simulink library "foc_blocks"  (R2020b)
settings: Solver=ode45  StartTime=0.0  StopTime=10.0  RelTol=1e-3  EnableMultiTasking=on
values from neighbouring files (symbols this model uses):
  ClockFrequency = 100    [setup_DF_fixp16_alu_av.m]    (also in setup_sim_DF_fixp16_alu.m; setup_verify_DF_fixp16_alu.m)
  constfractionlengthIn = 10    [setup_DF_fixp16_alu_av.m]    (also in setup_sim_DF_fixp16_alu.m; setup_verify_DF_fixp16_alu.m)
  constwordlengthIn = 16    [setup_DF_fixp16_alu_av.m]    (also in setup_sim_DF_fixp16_alu.m; setup_verify_DF_fixp16_alu.m)
  DSPBASampleTime = FoldingFactor / (ClockFrequency * 1e6)    (= 5e-06)    [setup_DF_fixp16_alu_av.m]    (also in setup_sim_DF_fixp16_alu.m; setup_verify_DF_fixp16_alu.m)
  FoldingFactor = 500    [setup_DF_fixp16_alu_av.m]    (also in setup_sim_DF_fixp16_alu.m; setup_verify_DF_fixp16_alu.m)
undefined symbols (not defined in the file or in its folder): AdvDSPBChannelOutDisplay, dpoly, dspba_ChannelInVis, dspba_ChannelOutVis, dspba_internal_get_channel_ports, evalAionMaskParam, latency, primtype, value, x
libraries: DSPBAPrim x559, AlteraGenericMotorLibrary x20, $bdroot x9, DSPBAUtilities x4, DSPBAControl x4
(part 2 of 6)

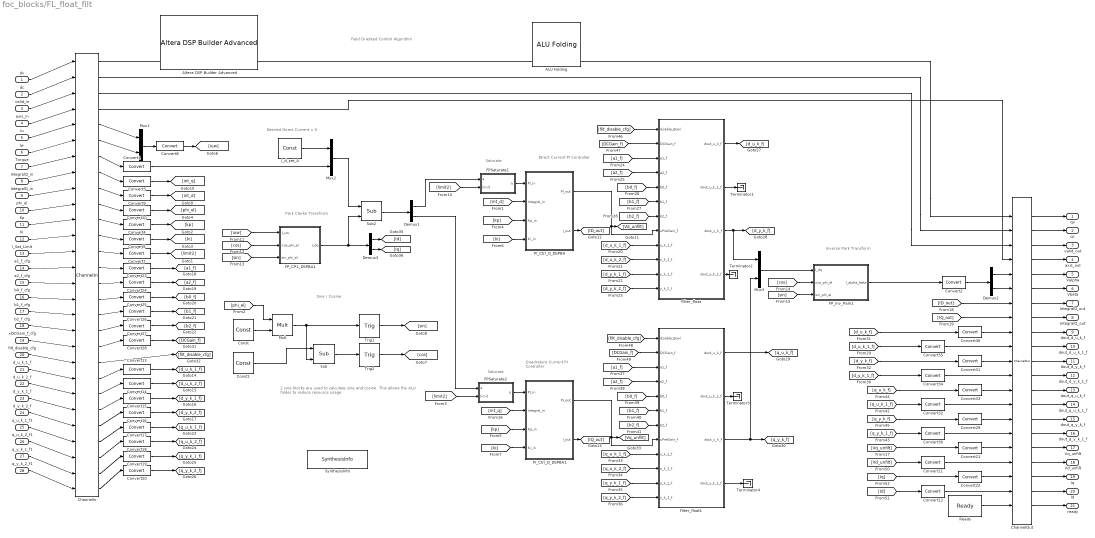
== system foc_blocks/FL_float_filt ==
  note: Quadrature Current
      | PI Controller
  note: Direct Current
      | PI Controller
  note: Desired Direct Current = 0
  note: Inverse Park
      |  Transform
  note: Park Clarke
      |  Transform
  note: Saturate
  note: Saturate
  note: Field Oriented Control Algorithm
  note: Sine / Cosine
  note: 2 sine blocks are used to calculate sine and cosine.
      | This allows the ALU folder to reduce resource usage.
  dv : Inport
  dc : Inport  Port=2
  valid_in : Inport  Port=3
  axis_in : Inport  Port=4
  Iu : Inport  Port=5
  Iw : Inport  Port=6
  Torque : Inport  Port=7
  IntegralQ_in : Inport  Port=8
  IntegralD_in : Inport  Port=9
  phi_el : Inport  Port=10
  Kp : Inport  Port=11
  Ki : Inport  Port=12
  I_Sat_Limit : Inport  Port=13
  a1_f_cfg : Inport  Port=14
  a2_f_cfg : Inport  Port=15
  b0_f_cfg : Inport  Port=16
  b1_f_cfg : Inport  Port=17
  b2_f_cfg : Inport  Port=18
  xDCGain_f_cfg : Inport  Port=19
  filt_disable_cfg : Inport  Port=20
  d_u_k_1_f : Inport  Port=21
  d_u_k_2_f : Inport  Port=22
  d_y_k_1_f : Inport  Port=23
  d_y_k_2_f : Inport  Port=24
  q_u_k_1_f1 : Inport  Port=25
  q_u_k_2_f1 : Inport  Port=26
  q_y_k_1_f1 : Inport  Port=27
  q_y_k_2_f1 : Inport  Port=28
  ALU Folding : DSPBAUtilities/ALU Folding  Description=Enables the new folder. When this block is placed in a subsystem, all primitive subsystems at the level it is placed and below will be passed to the folder. DSP Builder will then generate folded subsystems which can be placed back into the existing design.  version=20130913  genModelFileName=folded_model.xml  sampleRate=SampleRate  numChannels=1  maxLatency=LatencyConstraint  inputFormat=Parallel  outputFormat=Parallel  latchOutputs=off  originalRate=off  hasIdleState=off  padInputs=off  simRate=Clock rate
  Altera DSP Builder Advanced : AlteraGenericMotorLibrary/FP_Cur_Ctrl_DSPBA/Altera DSP Builder Advanced  SystemSampleTime=-1  VariantActivationTime=update diagram  Latency=0  AutoFrameSizeCalculation=off
  ChannelIn : DSPBAPrim/ChannelIn  primtype=channelin  nInputs=dspba_internal_get_channel_ports(gcb)  nOutputs=dspba_internal_get_channel_ports(gcb)  omode=Inherit via internal rule  otype=sfix(16)  scale=2^-15  rndmethod=Unbiased  factor=1  satmethod=Symmetric  shift_vec=[0 1 2 -1]  value=26  inPortNames=['v'; 'c'; '0'; '1'; '2'; '3'; '4'; '5'; '6'; '7'; '8'; '9'; 'A'; 'B'; 'D'; 'E'; 'F'; 'G'; 'H'; 'I'; 'J'; 'K'; 'L'; 'M'; 'N'; 'O'; 'P'; 'Q'; 'R'; 'S'; 'T'; 'U'; 'W'; 'X'; 'Y'; 'Z']  outPortNames=['v'; 'c'; '0'; '1'; '2'; '3'; '4'; '5'; '6'; '7'; '8'; '9'; 'A'; 'B'; 'D'; 'E'; 'F'; 'G'; 'H'; 'I'; 'J'; 'K'; 'L'; 'M'; 'N'; 'O'; 'P'; 'Q'; 'R'; 'S'; 'T'; 'U'; 'W'; 'X'; 'Y'; 'Z']  dspbaimage=dspba_prim.jpg  text=fprintf('In');  style=Optimised  dataSignals=26  foldingEnabled=off  channels=1  sampleRate=ClockFrequency/FoldingFactor  packetBeginPresent=off  packetBeginEnabled=off  visibilities=dspba_ChannelInVis(gcb)  latencyCorrection=0  scheduleOrigin=off  version=20141013
  ChannelOut : DSPBAPrim/ChannelOut  primtype=channelout  nInputs=dspba_internal_get_channel_ports(gcb)  nOutputs=dspba_internal_get_channel_ports(gcb)  omode=Inherit via internal rule  otype=sfix(16)  scale=2^-15  rndmethod=Unbiased  factor=1  satmethod=Symmetric  shift_vec=[0 1 2 -1]  value=19  inPortNames=['v'; 'c'; '0'; '1'; '2'; '3'; '4'; '5'; '6'; '7'; '8'; '9'; 'A'; 'B'; 'D'; 'E'; 'F'; 'G'; 'H'; 'I'; 'J'; 'K'; 'L'; 'M'; 'N'; 'O'; 'P'; 'Q'; 'R'; 'S'; 'T'; 'U'; 'W'; 'X'; 'Y'; 'Z']  outPortNames=['v'; 'c'; '0'; '1'; '2'; '3'; '4'; '5'; '6'; '7'; '8'; '9'; 'A'; 'B'; 'D'; 'E'; 'F'; 'G'; 'H'; 'I'; 'J'; 'K'; 'L'; 'M'; 'N'; 'O'; 'P'; 'Q'; 'R'; 'S'; 'T'; 'U'; 'W'; 'X'; 'Y'; 'Z']  dspbaimage=dspba_prim.jpg  text=fprintf('Out%s', AdvDSPBChannelOutDisplay(latency));  style=Optimised  dataSignals=19  foldingEnabled=off  channels=1  sampleRate=ClockFrequency/FoldingFactor  packetBeginPresent=off  packetBeginEnabled=off  visibilities=dspba_ChannelOutVis(gcb)  latency=173  latencyCorrection=0  version=20141013
  Const : DSPBAPrim/Const  primtype=const  nInputs=0  nOutputs=1  omode=Specify via dialog  otype=fpDT  scale=1  rndmethod=Unbiased  factor=1  satmethod=Symmetric  shift_vec=[0 1 2 -1]  value=2  inPortNames=['+'; '+';]  outPortNames=[' ']  dspbaimage=dspba_prim.jpg  text=fprintf('%s', num2str(value));  style=Optimised  visibilities=8 + 1024  floatPrecision=float26_m17  version=20120820
  Const1 : DSPBAPrim/Const  primtype=const  nInputs=0  nOutputs=1  omode=Specify via dialog  otype=fpDT  scale=1  rndmethod=Unbiased  factor=1  satmethod=Symmetric  shift_vec=[0 1 2 -1]  value=1/2  inPortNames=['+'; '+';]  outPortNames=[' ']  dspbaimage=dspba_prim.jpg  text=fprintf('%s', num2str(value));  style=Optimised  visibilities=8 + 1024  floatPrecision=float26_m17  version=20120820
  Convert{1,3..5,7..10,13..20,23..28} (22 alike) : DSPBAPrim/Convert  primtype=convert  nInputs=1  nOutputs=1  omode=Specify via dialog  otype=fpDT  scale=1  rndmethod=Unbiased  factor=1  satmethod=None  shift_vec=[0 1 2 -1]  value=round([0:255]/17)  inPortNames=[' '; ' ';]  outPortNames=[' '; 'c']  dspbaimage=dspba_prim.jpg  text=fprintf('convert');  style=Optimised  visibilities=8+64+256  clipdetect=off  floatPrecision=float32_m23  advOptions=[]  version=20130211
  Convert{2,11..12,21..22,29..36} (13 alike) : DSPBAPrim/Convert  primtype=convert  nInputs=1  nOutputs=1  omode=single  otype=constOType  scale=constScale  rndmethod=Truncate  factor=1  satmethod=None  shift_vec=[0 1 2 -1]  value=round([0:255]/17)  inPortNames=[' '; ' ';]  outPortNames=[' '; 'c']  dspbaimage=dspba_prim.jpg  text=fprintf('convert');  style=Optimised  visibilities=8+64+256  clipdetect=off  floatPrecision=float32_m23  advOptions=[]  version=20130211
  Demux1 : Demux  Outputs=2
  Demux2 : Demux  Outputs=2
  Demux3 : Demux  Outputs=2
  FPSaturate1 : Subsystem
      mask Display: color('w');fprintf('FP Var Sat\n');port_label('input',1,'a');port_label('input',2,'limit');port_label('output',1,'q');
  FPSaturate2 : Subsystem
      mask Display: color('w');fprintf('FP Var Sat\n');port_label('input',1,'a');port_label('input',2,'limit');port_label('output',1,'q');
  FP_CP1_DSPBA1 : Subsystem  Description=Clarke & Park Transforms
  FP_Inv_Park1 : Subsystem  Description=Inverse Park & Clarke transforms
  Filter_float : Subsystem
  Filter_float1 : Subsystem
  I_d_set_A : DSPBAPrim/Const  primtype=const  nInputs=0  nOutputs=1  omode=Specify via dialog  otype=fpDT  scale=1  rndmethod=Unbiased  factor=1  satmethod=Symmetric  shift_vec=[0 1 2 -1]  value=0  inPortNames=['+'; '+';]  outPortNames=[' ']  dspbaimage=dspba_prim.jpg  text=fprintf('%s', num2str(value));  style=Optimised  visibilities=8 + 1024  floatPrecision=float32_m23  version=20120820
  Mult : DSPBAPrim/Mult  primtype=mult  nInputs=2  nOutputs=1  omode=Inherit via internal rule  otype=sfix(16)  scale=2^-15  rndmethod=Unbiased  factor=1  satmethod=Symmetric  shift_vec=[0 1 2 -1]  value=0  inPortNames=[' '; ' ';]  outPortNames=[' ']  dspbaimage=dspba_prim.jpg  text=fprintf('X');  style=Optimised  visibilities=8+2^18+2^19  floatPrecision=float32_m23  floatRounding=faithful  advOptions=[]  version=20130115
  Mux1 : Mux  Inputs=2
  Mux2 : Mux  Inputs=2
  Mux3 : Mux  Inputs=2
  PI_Ctrl_D_DSPBA : Subsystem
  PI_Ctrl_D_DSPBA1 : Subsystem
  Ready : DSPBAPrim/Ready  primtype=ready  nInputs=0  nOutputs=1  omode=Inherit via internal rule  otype=ufix(1)  scale=2^-0  rndmethod=Unbiased  factor=1  satmethod=Asymmetric  shift_vec=[]  value=1  inPortNames=['']  outPortNames=[' ']  dspbaimage=dspba_prim.jpg  text=fprintf('Ready');  style=Processor  visibilities=0  floatPrecision=float32_m23  version=20131024
  Sub : DSPBAPrim/Sub  primtype=sub  nInputs=2  nOutputs=1  omode=Inherit via internal rule  otype=sfix(16)  scale=2^-15  rndmethod=Unbiased  factor=1  satmethod=Symmetric  shift_vec=[0 1 2 -1]  value=0  inPortNames=['+'; '-';]  outPortNames=[' ']  dspbaimage=dspba_prim.jpg  text=fprintf('-');  style=Optimised  visibilities=8+2^17+2^18  floatRounding=faithful  advOptions=[]  version=20130115
  Sub2 : DSPBAPrim/Sub  primtype=sub  nInputs=2  nOutputs=1  omode=Inherit via internal rule  otype=sfix(16)  scale=2^-15  rndmethod=Unbiased  factor=1  satmethod=Symmetric  shift_vec=[0 1 2 -1]  value=0  inPortNames=['+'; '-';]  outPortNames=[' ']  dspbaimage=dspba_prim.jpg  text=fprintf('-');  style=Optimised  visibilities=8  floatRounding=faithful  advOptions=[]  version=20130115
  SynthesisInfo : DSPBAPrim/SynthesisInfo  primtype=synthinfo  nInputs=0  nOutputs=0  omode=Inherit via internal rule  otype=sfix(16)  scale=2^-15  rndmethod=Truncate  factor=1  satmethod=Symmetric  shift_vec=[0 1 2 -1]  value=99  inPortNames=[' '; ' ';]  outPortNames=[' ']  dspbaimage=dspba_prim_ctrl.jpg  text=fprintf('Style=%s', style);  style=Scheduled  visibilities=32768  constraintInUse=off  constraintRelation=>  constraintLimit=2  bitAccurate=off  version=20150220
  Terminator{1..4} (4 alike) : Terminator
  Trig1 : DSPBAPrim/Trig  primtype=trigfunc  nInputs=1  nOutputs=1  omode=Inherit via internal rule  otype=sfix(16)  scale=2^-15  rndmethod=Unbiased  factor=1  satmethod=Symmetric  shift_vec=[0 1 2 -1]  value=round([0:255]/17)  inPortNames=[' '; ' ';]  outPortNames=[' ']  dspbaimage=dspba_prim_float.jpg  text=fprintf('sin(a)');  style=Optimised  visibilities=2^17+2^18  functionExpr=sin(pi*x)  advOptions=[]  version=20140803
  Trig2 : DSPBAPrim/Trig  primtype=trigfunc  nInputs=1  nOutputs=1  omode=Inherit via internal rule  otype=sfix(16)  scale=2^-15  rndmethod=Unbiased  factor=1  satmethod=Symmetric  shift_vec=[0 1 2 -1]  value=round([0:255]/17)  inPortNames=[' '; ' ';]  outPortNames=[' ']  dspbaimage=dspba_prim_float.jpg  text=fprintf('sin(a)');  style=Optimised  visibilities=2^17+2^18  functionExpr=sin(pi*x)  advOptions=[]  version=20140803
  qv : Outport
  qc : Outport  Port=2
  valid_out : Outport  Port=3
  axis_out : Outport  Port=4
  Valpha : Outport  Port=5
  Vbeta : Outport  Port=6
  IntegralD_out : Outport  Port=7
  IntegralQ_out : Outport  Port=8
  dout_d_u_k_f : Outport  Port=9
  dout_d_u_k_1_f : Outport  Port=10
  dout_d_y_k_f : Outport  Port=11
  dout_d_y_k_1_f : Outport  Port=12
  dout_q_u_k_f : Outport  Port=13
  dout_q_u_k_1_f : Outport  Port=14
  dout_q_y_k_f : Outport  Port=15
  dout_q_y_k_1_f : Outport  Port=16
  Vq_unfilt : Outport  Port=17
  Vd_unfilt : Outport  Port=18
  Iq : Outport  Port=19
  Id : Outport  Port=20
  ready : Outport  Port=21
  wires:
  ChannelIn/1 -> ChannelOut/1
  ChannelIn/2 -> ChannelOut/2
  ChannelIn/5 -> Mux1/1
  ChannelIn/6 -> Mux1/2
  ChannelIn/3 -> ChannelOut/3
  ChannelIn/7 -> Convert1/1
  FPSaturate2/1(q) -> PI_Ctrl_D_DSPBA1/1(PI_in)
  FPSaturate1/1(q) -> PI_Ctrl_D_DSPBA/1(PI_in)
  Mux3/1 -> FP_Inv_Park1/1(I_dq)
  FP_Inv_Park1/1(I_alpha_beta) -> Convert2/1
  Demux2/1 -> ChannelOut/5
  Demux2/2 -> ChannelOut/6
  I_d_set_A/1 -> Mux2/1
  Mux2/1 -> Sub2/1
  Sub2/1 -> Demux1/1
  Demux1/1 -> FPSaturate1/1(a)
  Demux1/2 -> FPSaturate2/1(a)
  ChannelIn/8 -> Convert3/1
  ChannelIn/9 -> Convert9/1
  ChannelIn/10 -> Convert10/1
  ChannelIn/11 -> Convert4/1
  ChannelIn/12 -> Convert5/1
  [int_q] -> PI_Ctrl_D_DSPBA1/2(Integral_in)
  [kp] -> PI_Ctrl_D_DSPBA1/3(Kp_in)
  [ki] -> PI_Ctrl_D_DSPBA1/4(Ki_in)
  [limit2] -> FPSaturate2/2(limit)
  [int_d] -> PI_Ctrl_D_DSPBA/2(Integral_in)
  [kp] -> PI_Ctrl_D_DSPBA/3(Kp_in)
  [ki] -> PI_Ctrl_D_DSPBA/4(Ki_in)
  [limit2] -> FPSaturate1/2(limit)
  [iuw] -> FP_CP1_DSPBA1/1(I_uw)
  [cos] -> FP_CP1_DSPBA1/2(cos_phi_el)
  [sin] -> FP_CP1_DSPBA1/3(sin_phi_el)
  Mux1/1 -> Convert8/1
  [cos] -> FP_Inv_Park1/2(cos_phi_el)
  [sin] -> FP_Inv_Park1/3(sin_phi_el)
  Convert7/1 -> [limit2]
  Convert5/1 -> [ki]
  Convert4/1 -> [kp]
  Convert8/1 -> [iuw]
  Convert1/1 -> Mux2/2
  ChannelIn/4 -> ChannelOut/4
  Convert2/1 -> Demux2/1
  [ID_out] -> ChannelOut/7
  PI_Ctrl_D_DSPBA/2(I_out) -> [ID_out]
  [IQ_out] -> ChannelOut/8
  PI_Ctrl_D_DSPBA1/2(I_out) -> [IQ_out]
  Filter_float/3(dout_y_k_f) -> [d_y_k_f], Mux3/1
  PI_Ctrl_D_DSPBA/1(PI_out) -> Filter_float/8(uPreGain_f), [Vd_unfilt]
  [d_u_k_1_f] -> Filter_float/9(u_k_1_f)
  [d_u_k_2_f] -> Filter_float/10(u_k_2_f)
  [d_y_k_1_f] -> Filter_float/11(y_k_1_f)
  [d_y_k_2_f] -> Filter_float/12(y_k_2_f)
  [b2_f] -> Filter_float/7(b2_f)
  [b1_f] -> Filter_float/6(b1_f)
  [b0_f] -> Filter_float/5(b0_f)
  [a2_f] -> Filter_float/4(a2_f)
  [a1_f] -> Filter_float/3(a1_f)
  Filter_float1/3(dout_y_k_f) -> [q_y_k_f], Mux3/2
  PI_Ctrl_D_DSPBA1/1(PI_out) -> Filter_float1/8(uPreGain_f), [Vq_unfilt]
  [q_u_k_1_f] -> Filter_float1/9(u_k_1_f)
  [q_u_k_2_f] -> Filter_float1/10(u_k_2_f)
  [q_y_k_1_f] -> Filter_float1/11(y_k_1_f)
  [q_y_k_2_f] -> Filter_float1/12(y_k_2_f)
  [b2_f] -> Filter_float1/7(b2_f)
  [b1_f] -> Filter_float1/6(b1_f)
  [b0_f] -> Filter_float1/5(b0_f)
  [a2_f] -> Filter_float1/4(a2_f)
  [a1_f] -> Filter_float1/3(a1_f)
  Filter_float/1(dout_u_k_f) -> [d_u_k_f]
  Filter_float/2(dout_u_k_1_f) -> Terminator1/1
  Filter_float/4(dout_y_k_1_f) -> Terminator2/1
  [filt_disable_cfg] -> Filter_float/1(disable_Bool)
  [DCGain_f] -> Filter_float/2(DCGain_f)
  Filter_float1/4(dout_y_k_1_f) -> Terminator4/1
  Filter_float1/2(dout_u_k_1_f) -> Terminator3/1
  Filter_float1/1(dout_u_k_f) -> [q_u_k_f]
  [filt_disable_cfg] -> Filter_float1/1(disable_Bool)
  [DCGain_f] -> Filter_float1/2(DCGain_f)
  [Vq_unfilt] -> Convert21/1
  [Vd_unfilt] -> Convert11/1
  Ready/1 -> ChannelOut/21
  FP_CP1_DSPBA1/1(I_dq) -> Demux3/1, Sub2/2
  Demux3/1 -> [Id]
  Demux3/2 -> [Iq]
  [Iq] -> Convert22/1
  [Id] -> Convert12/1
  [phi_el] -> Mult/1
  Const/1 -> Mult/2
  Const1/1 -> Sub/1
  Mult/1 -> Trig1/1, Sub/2
  Sub/1 -> Trig2/1
  Trig1/1 -> [sin]
  Trig2/1 -> [cos]
  Convert3/1 -> [int_q]
  Convert9/1 -> [int_d]
  Convert10/1 -> [phi_el]
  Convert22/1 -> ChannelOut/19
  Convert12/1 -> ChannelOut/20
  Convert11/1 -> ChannelOut/18
  Convert21/1 -> ChannelOut/17
  [q_y_k_f] -> Convert29/1
  [d_y_k_f] -> Convert31/1
  Convert23/1 -> [a1_f]
  Convert24/1 -> [a2_f]
  Convert25/1 -> [b0_f]
  Convert26/1 -> [b1_f]
  Convert27/1 -> [b2_f]
  Convert28/1 -> [DCGain_f]
  Convert13/1 -> [d_u_k_1_f]
  Convert14/1 -> [d_u_k_2_f]
  Convert15/1 -> [d_y_k_1_f]
  Convert16/1 -> [d_y_k_2_f]
  Convert17/1 -> [q_u_k_1_f]
  Convert18/1 -> [q_u_k_2_f]
  Convert19/1 -> [q_y_k_1_f]
  Convert20/1 -> [q_y_k_2_f]
  Convert29/1 -> ChannelOut/15
  [q_u_k_f] -> Convert33/1
  Convert31/1 -> ChannelOut/11
  [d_u_k_f] -> Convert36/1
  [q_y_k_1_f] -> Convert30/1
  [q_u_k_1_f] -> Convert32/1
  [d_y_k_1_f] -> Convert34/1
  [d_u_k_1_f] -> Convert35/1
  Convert30/1 -> ChannelOut/16
  Convert32/1 -> ChannelOut/14
  Convert33/1 -> ChannelOut/13
  Convert34/1 -> ChannelOut/12
  Convert35/1 -> ChannelOut/10
  Convert36/1 -> ChannelOut/9
  dv/1 -> ChannelIn/1
  dc/1 -> ChannelIn/2
  valid_in/1 -> ChannelIn/3
  axis_in/1 -> ChannelIn/4
  Iu/1 -> ChannelIn/5
  Iw/1 -> ChannelIn/6
  Torque/1 -> ChannelIn/7
  IntegralQ_in/1 -> ChannelIn/8
  IntegralD_in/1 -> ChannelIn/9
  phi_el/1 -> ChannelIn/10
  Kp/1 -> ChannelIn/11
  Ki/1 -> ChannelIn/12
  ChannelOut/1 -> qv/1
  ChannelOut/2 -> qc/1
  ChannelOut/3 -> valid_out/1
  ChannelOut/4 -> axis_out/1
  ChannelOut/5 -> Valpha/1
  ChannelOut/6 -> Vbeta/1
  ChannelOut/7 -> IntegralD_out/1
  ChannelOut/8 -> IntegralQ_out/1
  ChannelOut/9 -> dout_d_u_k_f/1
  ChannelOut/10 -> dout_d_u_k_1_f/1
  ChannelOut/11 -> dout_d_y_k_f/1
  ChannelOut/12 -> dout_d_y_k_1_f/1
  ChannelOut/13 -> dout_q_u_k_f/1
  ChannelOut/14 -> dout_q_u_k_1_f/1
  ChannelOut/15 -> dout_q_y_k_f/1
  ChannelOut/16 -> dout_q_y_k_1_f/1
  ChannelOut/17 -> Vq_unfilt/1
  ChannelOut/18 -> Vd_unfilt/1
  ChannelOut/19 -> Iq/1
  ChannelOut/20 -> Id/1
  ChannelOut/21 -> ready/1
  I_Sat_Limit/1 -> ChannelIn/13
  a1_f_cfg/1 -> ChannelIn/14
  a2_f_cfg/1 -> ChannelIn/15
  b0_f_cfg/1 -> ChannelIn/16
  b1_f_cfg/1 -> ChannelIn/17
  b2_f_cfg/1 -> ChannelIn/18
  xDCGain_f_cfg/1 -> ChannelIn/19
  filt_disable_cfg/1 -> ChannelIn/20
  d_u_k_1_f/1 -> ChannelIn/21
  d_u_k_2_f/1 -> ChannelIn/22
  d_y_k_1_f/1 -> ChannelIn/23
  d_y_k_2_f/1 -> ChannelIn/24
  q_u_k_1_f1/1 -> ChannelIn/25
  q_u_k_2_f1/1 -> ChannelIn/26
  q_y_k_1_f1/1 -> ChannelIn/27
  q_y_k_2_f1/1 -> ChannelIn/28
  ChannelIn/13 -> Convert7/1
  ChannelIn/14 -> Convert23/1
  ChannelIn/15 -> Convert24/1
  ChannelIn/16 -> Convert25/1
  ChannelIn/17 -> Convert26/1
  ChannelIn/18 -> Convert27/1
  ChannelIn/19 -> Convert28/1
  ChannelIn/20 -> [filt_disable_cfg]
  ChannelIn/21 -> Convert13/1
  ChannelIn/22 -> Convert14/1
  ChannelIn/23 -> Convert15/1
  ChannelIn/24 -> Convert16/1
  ChannelIn/25 -> Convert17/1
  ChannelIn/26 -> Convert18/1
  ChannelIn/27 -> Convert19/1
  ChannelIn/28 -> Convert20/1

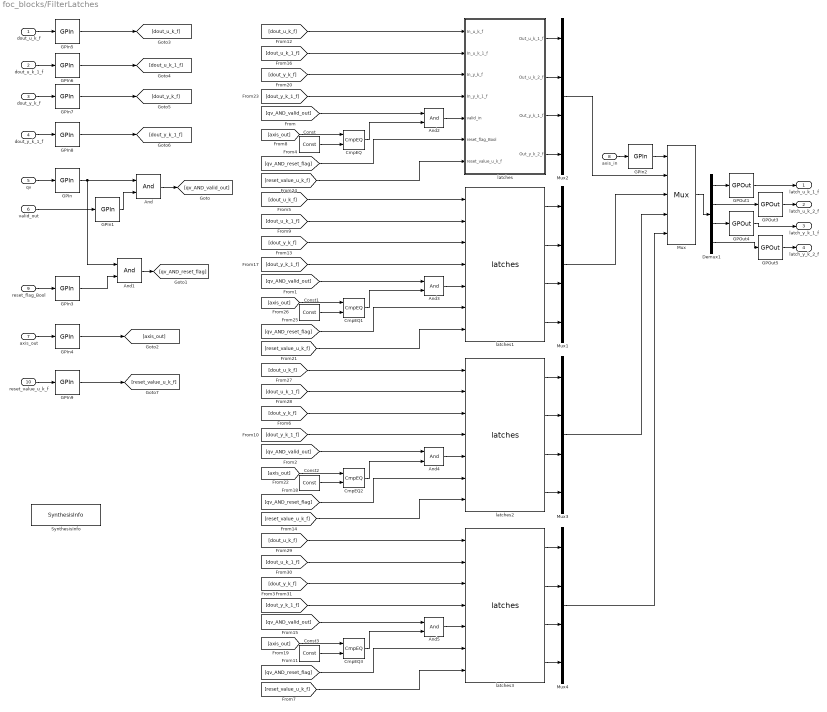
== system foc_blocks/FilterLatches ==
  dout_u_k_f : Inport
  dout_u_k_1_f : Inport  Port=2
  dout_y_k_f : Inport  Port=3
  dout_y_k_1_f : Inport  Port=4
  qv : Inport  Port=5
  valid_out : Inport  Port=6
  axis_out : Inport  Port=7
  axis_in : Inport  Port=8
  reset_flag_Bool : Inport  Port=9
  reset_value_u_k_f : Inport  Port=10
  And{,1..5} (6 alike) : DSPBAPrim/And  primtype=and  nInputs=2  nOutputs=1  omode=Inherit via internal rule  otype=sfix(16)  scale=2^-15  rndmethod=Unbiased  factor=1  satmethod=Symmetric  shift_vec=[0 1 2 -1]  value=0  inPortNames=[' '; ' '; ' '; ' '; ' '; ' '; ' '; ' '; ' '; ' '; ' '; ' '; ' '; ' '; ' '; ' '; ]  outPortNames=[' ']  dspbaimage=dspba_prim.jpg  text=fprintf('&');  style=Optimised  visibilities=8+2  version=20090407
  CmpEQ{,1..3} (4 alike) : DSPBAPrim/CmpEQ  primtype=cmpeq  nInputs=2  nOutputs=1  omode=boolean  otype=sfix(16)  scale=2^-15  rndmethod=Unbiased  factor=1  satmethod=Symmetric  shift_vec=[0 1 2 -1]  value=0  inPortNames=[' '; ' ';]  outPortNames=[' ']  dspbaimage=dspba_prim.jpg  text=fprintf('==');  style=Optimised  visibilities=0  advOptions=[]  version=20130117
  Const : DSPBAPrim/Const  primtype=const  nInputs=0  nOutputs=1  omode=Specify via dialog  otype=ufix(2)  scale=1  rndmethod=Unbiased  factor=1  satmethod=Symmetric  shift_vec=[0 1 2 -1]  value=0  inPortNames=['+'; '+';]  outPortNames=[' ']  dspbaimage=dspba_prim.jpg  text=fprintf('%s', num2str(value));  style=Optimised  visibilities=8 + 1024  floatPrecision=float32_m23  version=20120820
  Const1 : DSPBAPrim/Const  primtype=const  nInputs=0  nOutputs=1  omode=Specify via dialog  otype=ufix(2)  scale=1  rndmethod=Unbiased  factor=1  satmethod=Symmetric  shift_vec=[0 1 2 -1]  value=1  inPortNames=['+'; '+';]  outPortNames=[' ']  dspbaimage=dspba_prim.jpg  text=fprintf('%s', num2str(value));  style=Optimised  visibilities=8 + 1024  floatPrecision=float32_m23  version=20120820
  Const2 : DSPBAPrim/Const  primtype=const  nInputs=0  nOutputs=1  omode=Specify via dialog  otype=ufix(2)  scale=1  rndmethod=Unbiased  factor=1  satmethod=Symmetric  shift_vec=[0 1 2 -1]  value=2  inPortNames=['+'; '+';]  outPortNames=[' ']  dspbaimage=dspba_prim.jpg  text=fprintf('%s', num2str(value));  style=Optimised  visibilities=8 + 1024  floatPrecision=float32_m23  version=20120820
  Const3 : DSPBAPrim/Const  primtype=const  nInputs=0  nOutputs=1  omode=Specify via dialog  otype=ufix(2)  scale=1  rndmethod=Unbiased  factor=1  satmethod=Symmetric  shift_vec=[0 1 2 -1]  value=3  inPortNames=['+'; '+';]  outPortNames=[' ']  dspbaimage=dspba_prim.jpg  text=fprintf('%s', num2str(value));  style=Optimised  visibilities=8 + 1024  floatPrecision=float32_m23  version=20120820
  Demux1 : Demux
  GPIn{,1..9} (10 alike) : DSPBAPrim/GPIn  primtype=gpin  nInputs=evalAionMaskParam(gcb,'value',1)  nOutputs=evalAionMaskParam(gcb,'value',1)  omode=Inherit via internal rule  otype=sfix(16)  scale=2^-15  rndmethod=Unbiased  factor=1  satmethod=Symmetric  shift_vec=[0 1 2 -1]  value=1  inPortNames=[' ' ' ' ' ' ' ' ' ' ' ' ' ' ' ' ' ' ' ' ' ' ' ' ' ' ' ' ' ' ' ' ' ' ' ' ' ' ' ' ' ' ' ' ' ' ' ' ' ' ' ' ' ' ' ' ' ' ' ' ' ' ' ' ' ' ' ' ' ']'  outPortNames=[' ' ' ' ' ' ' ' ' ' ' ' ' ' ' ' ' ' ' ' ' ' ' ' ' ' ' ' ' ' ' ' ' ' ' ' ' ' ' ' ' ' ' ' ' ' ' ' ' ' ' ' ' ' ' ' ' ' ' ' ' ' ' ' ' ' ' ' ' ']'  dspbaimage=dspba_prim.jpg  text=fprintf('GPIn');  style=Optimised  visibilities=1024  latencyCorrection=0  scheduleOrigin=off  version=20090407
  GPOut{1,3..5} (4 alike) : DSPBAPrim/GPOut  primtype=gpout  nInputs=evalAionMaskParam(gcb,'value',1)  nOutputs=evalAionMaskParam(gcb,'value',1)  omode=Inherit via internal rule  otype=sfix(16)  scale=2^-15  rndmethod=Unbiased  factor=1  satmethod=Symmetric  shift_vec=[0 1 2 -1]  value=1  inPortNames=[' ' ' ' ' ' ' ' ' ' ' ' ' ' ' ' ' ' ' ' ' ' ' ' ' ' ' ' ' ' ' ' ' ' ' ' ' ' ' ' ' ' ' ' ' ' ' ' ' ' ' ' ' ' ' ' ' ' ' ' ' ' ' ' ' ' ' ' ' ']'  outPortNames=[' ' ' ' ' ' ' ' ' ' ' ' ' ' ' ' ' ' ' ' ' ' ' ' ' ' ' ' ' ' ' ' ' ' ' ' ' ' ' ' ' ' ' ' ' ' ' ' ' ' ' ' ' ' ' ' ' ' ' ' ' ' ' ' ' ' ' ' ' ']'  dspbaimage=dspba_prim.jpg  text=fprintf('GPOut');  style=Optimised  visibilities=1024  latencyCorrection=0  version=20090407
  Mux : DSPBAPrim/Mux  primtype=mux  nInputs=evalAionMaskParam(gcb,'value',1)+1  nOutputs=1  omode=Inherit via internal rule  otype=sfix(16)  scale=2^-15  rndmethod=Unbiased  factor=1  satmethod=Symmetric  shift_vec=[0 1 2 -1]  value=4  inPortNames=['s'; 'd0'; 'd1'; 'd2'; 'd3'; 'd4'; 'd5'; 'd6'; 'd7'; 'd8'; 'd9';]  outPortNames=[' ']  dspbaimage=dspba_prim.jpg  text=fprintf('%s', primtype);  style=Optimised  visibilities=1032  version=20131025
  Mux{1..4} (4 alike) : Mux
  SynthesisInfo : DSPBAPrim/SynthesisInfo  primtype=synthinfo  nInputs=0  nOutputs=0  omode=Inherit via internal rule  otype=sfix(16)  scale=2^-15  rndmethod=Truncate  factor=1  satmethod=Symmetric  shift_vec=[0 1 2 -1]  value=99  inPortNames=[' '; ' ';]  outPortNames=[' ']  dspbaimage=dspba_prim_ctrl.jpg  text=fprintf('Style=%s', style);  style=Scheduled  visibilities=32768  constraintInUse=off  constraintRelation=>  constraintLimit=2  bitAccurate=off  version=20150220
  latches : Subsystem
  latches1 : $bdroot/FilterLatches/latches  SystemSampleTime=-1  VariantActivationTime=update diagram  Latency=0  AutoFrameSizeCalculation=off
  latches2 : $bdroot/FilterLatches/latches  SystemSampleTime=-1  VariantActivationTime=update diagram  Latency=0  AutoFrameSizeCalculation=off
  latches3 : $bdroot/FilterLatches/latches  SystemSampleTime=-1  VariantActivationTime=update diagram  Latency=0  AutoFrameSizeCalculation=off
  latch_u_k_1_f : Outport  SampleTime=DSPBASampleTime
  latch_u_k_2_f : Outport  Port=2  SampleTime=DSPBASampleTime
  latch_y_k_1_f : Outport  Port=3  SampleTime=DSPBASampleTime
  latch_y_k_2_f : Outport  Port=4  SampleTime=DSPBASampleTime
  wires:
  qv/1 -> GPIn/1
  valid_out/1 -> GPIn1/1
  reset_flag_Bool/1 -> GPIn3/1
  Const/1 -> CmpEQ/2
  CmpEQ/1 -> And2/2
  And2/1 -> latches/5(valid_in)
  latches/1(Out_u_k_1_f) -> Mux2/1
  latches/2(Out_u_k_2_f) -> Mux2/2
  Demux1/1 -> GPOut1/1
  Demux1/2 -> GPOut3/1
  Mux/1 -> Demux1/1
  Mux2/1 -> Mux/2
  axis_in/1 -> GPIn2/1
  latches/3(Out_y_k_1_f) -> Mux2/3
  latches/4(Out_y_k_2_f) -> Mux2/4
  axis_out/1 -> GPIn4/1
  [qv_AND_valid_out] -> And2/1
  And/1 -> [qv_AND_valid_out]
  And1/1 -> [qv_AND_reset_flag]
  [qv_AND_reset_flag] -> latches/6(reset_flag_Bool)
  reset_value_u_k_f/1 -> GPIn9/1
  [dout_u_k_1_f] -> latches/2(In_u_k_1_f)
  dout_y_k_f/1 -> GPIn7/1
  dout_y_k_1_f/1 -> GPIn8/1
  latches1/4 -> Mux1/4
  latches1/3 -> Mux1/3
  latches1/2 -> Mux1/2
  latches1/1 -> Mux1/1
  Mux1/1 -> Mux/3
  latches2/4 -> Mux3/4
  latches3/4 -> Mux4/4
  latches2/1 -> Mux3/1
  latches2/2 -> Mux3/2
  latches2/3 -> Mux3/3
  Mux3/1 -> Mux/4
  latches3/1 -> Mux4/1
  latches3/2 -> Mux4/2
  latches3/3 -> Mux4/3
  Mux4/1 -> Mux/5
  Demux1/3 -> GPOut4/1
  Demux1/4 -> GPOut5/1
  GPIn1/1 -> And/2
  GPIn/1 -> And1/1, And/1
  GPIn3/1 -> And1/2
  GPIn4/1 -> [axis_out]
  [axis_out] -> CmpEQ/1
  dout_u_k_f/1 -> GPIn5/1
  GPIn5/1 -> [dout_u_k_f]
  [dout_u_k_f] -> latches/1(In_u_k_f)
  dout_u_k_1_f/1 -> GPIn6/1
  GPIn6/1 -> [dout_u_k_1_f]
  GPIn7/1 -> [dout_y_k_f]
  [dout_y_k_f] -> latches/3(In_y_k_f)
  GPIn8/1 -> [dout_y_k_1_f]
  [dout_y_k_1_f] -> latches/4(In_y_k_1_f)
  GPIn9/1 -> [reset_value_u_k_f]
  [reset_value_u_k_f] -> latches/7(reset_value_u_k_f)
  Const1/1 -> CmpEQ1/2
  CmpEQ1/1 -> And3/2
  And3/1 -> latches1/5
  [qv_AND_valid_out] -> And3/1
  [qv_AND_reset_flag] -> latches1/6
  [dout_u_k_1_f] -> latches1/2
  [axis_out] -> CmpEQ1/1
  [dout_u_k_f] -> latches1/1
  [dout_y_k_f] -> latches1/3
  [dout_y_k_1_f] -> latches1/4
  [reset_value_u_k_f] -> latches1/7
  Const2/1 -> CmpEQ2/2
  CmpEQ2/1 -> And4/2
  And4/1 -> latches2/5
  [qv_AND_valid_out] -> And4/1
  [qv_AND_reset_flag] -> latches2/6
  [dout_u_k_1_f] -> latches2/2
  [axis_out] -> CmpEQ2/1
  [dout_u_k_f] -> latches2/1
  [dout_y_k_f] -> latches2/3
  [dout_y_k_1_f] -> latches2/4
  [reset_value_u_k_f] -> latches2/7
  Const3/1 -> CmpEQ3/2
  CmpEQ3/1 -> And5/2
  And5/1 -> latches3/5
  [qv_AND_valid_out] -> And5/1
  [qv_AND_reset_flag] -> latches3/6
  [dout_u_k_1_f] -> latches3/2
  [axis_out] -> CmpEQ3/1
  [dout_u_k_f] -> latches3/1
  [dout_y_k_f] -> latches3/3
  [dout_y_k_1_f] -> latches3/4
  [reset_value_u_k_f] -> latches3/7
  GPOut1/1 -> latch_u_k_1_f/1
  GPOut3/1 -> latch_u_k_2_f/1
  GPOut4/1 -> latch_y_k_1_f/1
  GPOut5/1 -> latch_y_k_2_f/1
  GPIn2/1 -> Mux/1

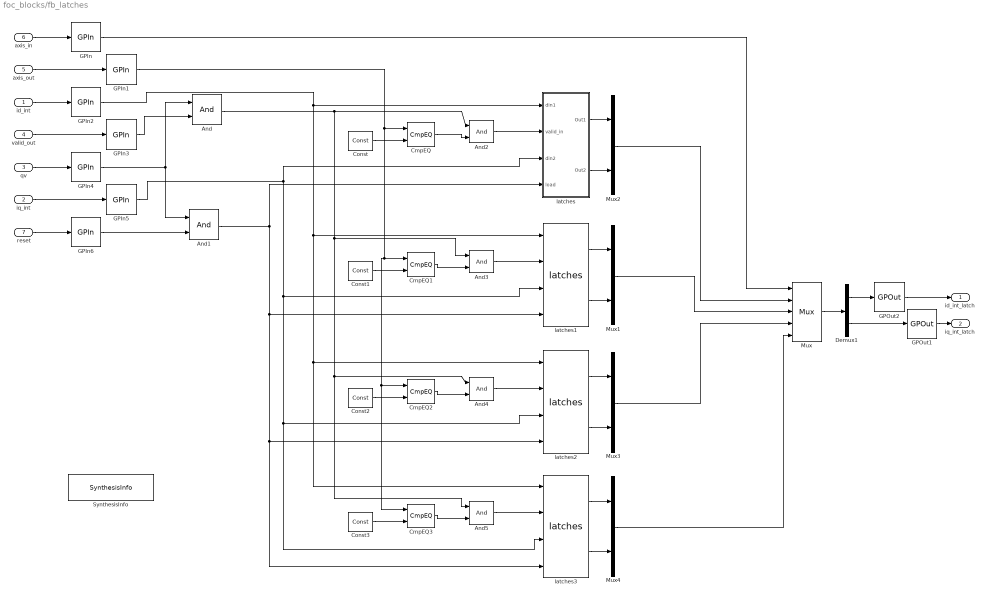
== system foc_blocks/fb_latches ==
  id_int : Inport
  iq_int : Inport  Port=2
  qv : Inport  Port=3
  valid_out : Inport  Port=4
  axis_out : Inport  Port=5
  axis_in : Inport  Port=6
  reset : Inport  Port=7
  And{,1..5} (6 alike) : DSPBAPrim/And  primtype=and  nInputs=2  nOutputs=1  omode=Inherit via internal rule  otype=sfix(16)  scale=2^-15  rndmethod=Unbiased  factor=1  satmethod=Symmetric  shift_vec=[0 1 2 -1]  value=0  inPortNames=[' '; ' '; ' '; ' '; ' '; ' '; ' '; ' '; ' '; ' '; ' '; ' '; ' '; ' '; ' '; ' '; ]  outPortNames=[' ']  dspbaimage=dspba_prim.jpg  text=fprintf('&');  style=Optimised  visibilities=8+2  version=20090407
  CmpEQ{,1..3} (4 alike) : DSPBAPrim/CmpEQ  primtype=cmpeq  nInputs=2  nOutputs=1  omode=boolean  otype=sfix(16)  scale=2^-15  rndmethod=Unbiased  factor=1  satmethod=Symmetric  shift_vec=[0 1 2 -1]  value=0  inPortNames=[' '; ' ';]  outPortNames=[' ']  dspbaimage=dspba_prim.jpg  text=fprintf('==');  style=Optimised  visibilities=0  advOptions=[]  version=20130117
  Const : DSPBAPrim/Const  primtype=const  nInputs=0  nOutputs=1  omode=Specify via dialog  otype=ufix(2)  scale=1  rndmethod=Unbiased  factor=1  satmethod=Symmetric  shift_vec=[0 1 2 -1]  value=0  inPortNames=['+'; '+';]  outPortNames=[' ']  dspbaimage=dspba_prim.jpg  text=fprintf('%s', num2str(value));  style=Optimised  visibilities=8 + 1024  floatPrecision=float32_m23  version=20120820
  Const1 : DSPBAPrim/Const  primtype=const  nInputs=0  nOutputs=1  omode=Specify via dialog  otype=ufix(2)  scale=1  rndmethod=Unbiased  factor=1  satmethod=Symmetric  shift_vec=[0 1 2 -1]  value=1  inPortNames=['+'; '+';]  outPortNames=[' ']  dspbaimage=dspba_prim.jpg  text=fprintf('%s', num2str(value));  style=Optimised  visibilities=8 + 1024  floatPrecision=float32_m23  version=20120820
  Const2 : DSPBAPrim/Const  primtype=const  nInputs=0  nOutputs=1  omode=Specify via dialog  otype=ufix(2)  scale=1  rndmethod=Unbiased  factor=1  satmethod=Symmetric  shift_vec=[0 1 2 -1]  value=2  inPortNames=['+'; '+';]  outPortNames=[' ']  dspbaimage=dspba_prim.jpg  text=fprintf('%s', num2str(value));  style=Optimised  visibilities=8 + 1024  floatPrecision=float32_m23  version=20120820
  Const3 : DSPBAPrim/Const  primtype=const  nInputs=0  nOutputs=1  omode=Specify via dialog  otype=ufix(2)  scale=1  rndmethod=Unbiased  factor=1  satmethod=Symmetric  shift_vec=[0 1 2 -1]  value=3  inPortNames=['+'; '+';]  outPortNames=[' ']  dspbaimage=dspba_prim.jpg  text=fprintf('%s', num2str(value));  style=Optimised  visibilities=8 + 1024  floatPrecision=float32_m23  version=20120820
  Demux1 : Demux  Outputs=2
  GPIn{,1..6} (7 alike) : DSPBAPrim/GPIn  primtype=gpin  nInputs=evalAionMaskParam(gcb,'value',1)  nOutputs=evalAionMaskParam(gcb,'value',1)  omode=Inherit via internal rule  otype=sfix(16)  scale=2^-15  rndmethod=Unbiased  factor=1  satmethod=Symmetric  shift_vec=[0 1 2 -1]  value=1  inPortNames=[' ' ' ' ' ' ' ' ' ' ' ' ' ' ' ' ' ' ' ' ' ' ' ' ' ' ' ' ' ' ' ' ' ' ' ' ' ' ' ' ' ' ' ' ' ' ' ' ' ' ' ' ' ' ' ' ' ' ' ' ' ' ' ' ' ' ' ' ' ']'  outPortNames=[' ' ' ' ' ' ' ' ' ' ' ' ' ' ' ' ' ' ' ' ' ' ' ' ' ' ' ' ' ' ' ' ' ' ' ' ' ' ' ' ' ' ' ' ' ' ' ' ' ' ' ' ' ' ' ' ' ' ' ' ' ' ' ' ' ' ' ' ' ']'  dspbaimage=dspba_prim.jpg  text=fprintf('GPIn');  style=Optimised  visibilities=1024  latencyCorrection=0  scheduleOrigin=off  version=20090407
  GPOut1 : DSPBAPrim/GPOut  primtype=gpout  nInputs=evalAionMaskParam(gcb,'value',1)  nOutputs=evalAionMaskParam(gcb,'value',1)  omode=Inherit via internal rule  otype=sfix(16)  scale=2^-15  rndmethod=Unbiased  factor=1  satmethod=Symmetric  shift_vec=[0 1 2 -1]  value=1  inPortNames=[' ' ' ' ' ' ' ' ' ' ' ' ' ' ' ' ' ' ' ' ' ' ' ' ' ' ' ' ' ' ' ' ' ' ' ' ' ' ' ' ' ' ' ' ' ' ' ' ' ' ' ' ' ' ' ' ' ' ' ' ' ' ' ' ' ' ' ' ' ']'  outPortNames=[' ' ' ' ' ' ' ' ' ' ' ' ' ' ' ' ' ' ' ' ' ' ' ' ' ' ' ' ' ' ' ' ' ' ' ' ' ' ' ' ' ' ' ' ' ' ' ' ' ' ' ' ' ' ' ' ' ' ' ' ' ' ' ' ' ' ' ' ' ']'  dspbaimage=dspba_prim.jpg  text=fprintf('GPOut');  style=Optimised  visibilities=1024  latencyCorrection=0  version=20090407
  GPOut2 : DSPBAPrim/GPOut  primtype=gpout  nInputs=evalAionMaskParam(gcb,'value',1)  nOutputs=evalAionMaskParam(gcb,'value',1)  omode=Inherit via internal rule  otype=sfix(16)  scale=2^-15  rndmethod=Unbiased  factor=1  satmethod=Symmetric  shift_vec=[0 1 2 -1]  value=1  inPortNames=[' ' ' ' ' ' ' ' ' ' ' ' ' ' ' ' ' ' ' ' ' ' ' ' ' ' ' ' ' ' ' ' ' ' ' ' ' ' ' ' ' ' ' ' ' ' ' ' ' ' ' ' ' ' ' ' ' ' ' ' ' ' ' ' ' ' ' ' ' ']'  outPortNames=[' ' ' ' ' ' ' ' ' ' ' ' ' ' ' ' ' ' ' ' ' ' ' ' ' ' ' ' ' ' ' ' ' ' ' ' ' ' ' ' ' ' ' ' ' ' ' ' ' ' ' ' ' ' ' ' ' ' ' ' ' ' ' ' ' ' ' ' ' ']'  dspbaimage=dspba_prim.jpg  text=fprintf('GPOut');  style=Optimised  visibilities=1024  latencyCorrection=0  version=20090407
  Mux : DSPBAPrim/Mux  primtype=mux  nInputs=evalAionMaskParam(gcb,'value',1)+1  nOutputs=1  omode=Inherit via internal rule  otype=sfix(16)  scale=2^-15  rndmethod=Unbiased  factor=1  satmethod=Symmetric  shift_vec=[0 1 2 -1]  value=4  inPortNames=['s'; 'd0'; 'd1'; 'd2'; 'd3'; 'd4'; 'd5'; 'd6'; 'd7'; 'd8'; 'd9';]  outPortNames=[' ']  dspbaimage=dspba_prim.jpg  text=fprintf('%s', primtype);  style=Optimised  visibilities=1032  version=20131025
  Mux{1..4} (4 alike) : Mux  Inputs=2
  SynthesisInfo : DSPBAPrim/SynthesisInfo  primtype=synthinfo  nInputs=0  nOutputs=0  omode=Inherit via internal rule  otype=sfix(16)  scale=2^-15  rndmethod=Truncate  factor=1  satmethod=Symmetric  shift_vec=[0 1 2 -1]  value=99  inPortNames=[' '; ' ';]  outPortNames=[' ']  dspbaimage=dspba_prim_ctrl.jpg  text=fprintf('Style=%s', style);  style=Scheduled  visibilities=32768  constraintInUse=off  constraintRelation=>  constraintLimit=2  bitAccurate=off  version=20150220
  latches : Subsystem
  latches1 : $bdroot/fb_latches/latches  SystemSampleTime=-1  VariantActivationTime=update diagram  Latency=0  AutoFrameSizeCalculation=off
  latches2 : $bdroot/fb_latches/latches  SystemSampleTime=-1  VariantActivationTime=update diagram  Latency=0  AutoFrameSizeCalculation=off
  latches3 : $bdroot/fb_latches/latches  SystemSampleTime=-1  VariantActivationTime=update diagram  Latency=0  AutoFrameSizeCalculation=off
  id_int_latch : Outport
  iq_int_latch : Outport  Port=2
  wires:
  And1/1 -> latches1/4, latches3/4, latches2/4, latches/4(load)
  Const/1 -> CmpEQ/2
  CmpEQ/1 -> And2/2
  And/1 -> And2/1, And5/1, And4/1, And3/1
  And2/1 -> latches/2(valid_in)
  latches/1(Out1) -> Mux2/1
  latches/2(Out2) -> Mux2/2
  Mux/1 -> Demux1/1
  Const1/1 -> CmpEQ1/2
  CmpEQ1/1 -> And3/2
  And3/1 -> latches1/2
  latches1/1 -> Mux1/1
  latches1/2 -> Mux1/2
  Const2/1 -> CmpEQ2/2
  CmpEQ2/1 -> And4/2
  And4/1 -> latches2/2
  latches2/1 -> Mux3/1
  latches2/2 -> Mux3/2
  Const3/1 -> CmpEQ3/2
  CmpEQ3/1 -> And5/2
  And5/1 -> latches3/2
  latches3/1 -> Mux4/1
  latches3/2 -> Mux4/2
  Mux2/1 -> Mux/2
  Mux1/1 -> Mux/3
  Mux3/1 -> Mux/4
  Mux4/1 -> Mux/5
  axis_in/1 -> GPIn/1
  axis_out/1 -> GPIn1/1
  id_int/1 -> GPIn2/1
  valid_out/1 -> GPIn3/1
  qv/1 -> GPIn4/1
  iq_int/1 -> GPIn5/1
  reset/1 -> GPIn6/1
  Demux1/1 -> GPOut2/1
  Demux1/2 -> GPOut1/1
  GPIn/1 -> Mux/1
  GPIn1/1 -> CmpEQ/1, CmpEQ1/1, CmpEQ2/1, CmpEQ3/1
  GPIn2/1 -> latches1/1, latches3/1, latches2/1, latches/1(din1)
  GPIn3/1 -> And/2
  GPIn4/1 -> And/1, And1/1
  GPIn5/1 -> latches1/3, latches3/3, latches2/3, latches/3(din2)
  GPIn6/1 -> And1/2
  GPOut2/1 -> id_int_latch/1
  GPOut1/1 -> iq_int_latch/1

== system foc_blocks/FL_fixp16/FP_CP1_DSPBA ==
  note: Sin/Cos Electrical Angle
  note: Feedback Current
  note: Park & Clarke Transform
  I_uw : Inport
  cos_phi_el : Inport  Port=2
  sin_phi_el : Inport  Port=3
  Add : DSPBAPrim/Add  primtype=add  nInputs=evalAionMaskParam(gcb,'value',1)  nOutputs=1  omode=Inherit via internal rule  otype=sfix(16)  scale=2^-15  rndmethod=Unbiased  factor=1  satmethod=Symmetric  shift_vec=[0 1 2 -1]  value=2  inPortNames=[' '; ' ';]  outPortNames=[' ']  dspbaimage=dspba_prim.jpg  text=fprintf('+');  style=Optimised  visibilities=1032  genFPC=off  floatRounding=correct  advOptions=[]  version=20130821
  Add1 : DSPBAPrim/Add  primtype=add  nInputs=evalAionMaskParam(gcb,'value',1)  nOutputs=1  omode=Inherit via internal rule  otype=sfix(16)  scale=2^-15  rndmethod=Unbiased  factor=1  satmethod=Symmetric  shift_vec=[0 1 2 -1]  value=2  inPortNames=[' '; ' ';]  outPortNames=[' ']  dspbaimage=dspba_prim.jpg  text=fprintf('+');  style=Optimised  visibilities=1032  genFPC=off  floatRounding=correct  advOptions=[]  version=20130821
  Altera DSP Builder Advanced : AlteraGenericMotorLibrary/FP_Cur_Ctrl_DSPBA/Altera DSP Builder Advanced  SystemSampleTime=-1  VariantActivationTime=update diagram  Latency=0  AutoFrameSizeCalculation=off
  Demux1 : Demux  Outputs=2
  FixedGain : Subsystem  mask{constVal=2}
      mask prompts: constVal "Gain"
      mask Display: color('w');fprintf('Fixed Gain\n%s', num2str(constVal));port_label('input',1,'a');port_label('output',1,'q');
  FixedGain1 : Subsystem  mask{constVal=-1/sqrt(3)}
      mask prompts: constVal "Gain"
      mask Display: color('w');fprintf('Fixed Gain\n%s', num2str(constVal));port_label('input',1,'a');port_label('output',1,'q');
  Mult{,1..3} (4 alike) : DSPBAPrim/Mult  primtype=mult  nInputs=2  nOutputs=1  omode=Specify via dialog  otype=constOTypeIn  scale=constScaleIn  rndmethod=Unbiased  factor=1  satmethod=Symmetric  shift_vec=[0 1 2 -1]  value=0  inPortNames=[' '; ' ';]  outPortNames=[' ']  dspbaimage=dspba_prim.jpg  text=fprintf('X');  style=Optimised  visibilities=8  floatPrecision=float32_m23  floatRounding=correct  advOptions=[]  version=20130115
  Mux1 : Mux  Inputs=2
  Sub1 : DSPBAPrim/Sub  primtype=sub  nInputs=2  nOutputs=1  omode=Inherit via internal rule  otype=sfix(16)  scale=2^-15  rndmethod=Unbiased  factor=1  satmethod=Symmetric  shift_vec=[0 1 2 -1]  value=0  inPortNames=['+'; '-';]  outPortNames=[' ']  dspbaimage=dspba_prim.jpg  text=fprintf('-');  style=Optimised  visibilities=8  floatRounding=correct  advOptions=[]  version=20130115
  I_dq : Outport
  wires:
  FixedGain/1(Out1) -> Add1/2
  Add1/1 -> FixedGain1/1(In1)
  sin_phi_el/1 -> Mult2/1, Mult1/2
  I_uw/1 -> Demux1/1
  Demux1/2 -> FixedGain/1(In1)
  Demux1/1 -> Add1/1, Mult/1, Mult2/2
  FixedGain1/1(Out1) -> Mult1/1, Mult3/1
  cos_phi_el/1 -> Mult3/2, Mult/2
  Mult/1 -> Add/1
  Mult1/1 -> Add/2
  Mult2/1 -> Sub1/2
  Mult3/1 -> Sub1/1
  Mux1/1 -> I_dq/1
  Add/1 -> Mux1/1
  Sub1/1 -> Mux1/2

== system foc_blocks/FL_fixp16/FP_Inv_Park ==
  note: Alpha/Beta Voltage
  note: Direct/Quadrature Voltage
  note: Sin/Cos Electrical Angle
  note: Inverse Park Transform
  V_dq : Inport
  cos_phi_el : Inport  Port=2
  sin_phi_el : Inport  Port=3
  Add : DSPBAPrim/Add  primtype=add  nInputs=evalAionMaskParam(gcb,'value',1)  nOutputs=1  omode=Inherit via internal rule with word growth  otype=constOTypeIn  scale=constScaleIn  rndmethod=Unbiased  factor=1  satmethod=Symmetric  shift_vec=[0 1 2 -1]  value=2  inPortNames=[' '; ' ';]  outPortNames=[' ']  dspbaimage=dspba_prim.jpg  text=fprintf('+');  style=Optimised  visibilities=1032  genFPC=off  floatRounding=correct  advOptions=[]  version=20130821
  Altera DSP Builder Advanced : AlteraGenericMotorLibrary/FP_Cur_Ctrl_DSPBA/Altera DSP Builder Advanced  SystemSampleTime=-1  VariantActivationTime=update diagram  Latency=0  AutoFrameSizeCalculation=off
  Demux1 : Demux  Outputs=2
  Mult{,1..3} (4 alike) : DSPBAPrim/Mult  primtype=mult  nInputs=2  nOutputs=1  omode=Specify via dialog  otype=constOTypeMult  scale=constScaleIn  rndmethod=Unbiased  factor=1  satmethod=Symmetric  shift_vec=[0 1 2 -1]  value=0  inPortNames=[' '; ' ';]  outPortNames=[' ']  dspbaimage=dspba_prim.jpg  text=fprintf('X');  style=Optimised  visibilities=8  floatPrecision=float32_m23  floatRounding=correct  advOptions=[]  version=20130115
  Mux2 : Mux  Inputs=2
  Sub1 : DSPBAPrim/Sub  primtype=sub  nInputs=2  nOutputs=1  omode=Inherit via internal rule with word growth  otype=constOTypeIn  scale=constScaleIn  rndmethod=Unbiased  factor=1  satmethod=Symmetric  shift_vec=[0 1 2 -1]  value=0  inPortNames=['+'; '-';]  outPortNames=[' ']  dspbaimage=dspba_prim.jpg  text=fprintf('-');  style=Optimised  visibilities=8  floatRounding=correct  advOptions=[]  version=20130115
  V_alpha_beta : Outport
  wires:
  Add/1 -> Mux2/2
  Sub1/1 -> Mux2/1
  Mux2/1 -> V_alpha_beta/1
  V_dq/1 -> Demux1/1
  sin_phi_el/1 -> Mult1/2, Mult2/2
  Demux1/2 -> Mult3/1, Mult1/1  "I_q"
  cos_phi_el/1 -> Mult/2, Mult3/2
  Demux1/1 -> Mult2/1, Mult/1  "I_d"
  Mult1/1 -> Sub1/2
  Mult/1 -> Sub1/1
  Mult3/1 -> Add/2
  Mult2/1 -> Add/1

== system foc_blocks/FL_fixp16/Fixed Saturate1 ==
  In1 : Inport
  limit : Inport  Port=2
  MinMax : DSPBAPrim/MinMax  primtype=minmaxfunc  nInputs=2  nOutputs=1  omode=Specify via dialog  otype=constOTypeIn  scale=constScaleIn  rndmethod=Unbiased  factor=1  satmethod=Symmetric  shift_vec=[0 1 2 -1]  value=0  inPortNames=[' '; ' ';]  outPortNames=[' ']  dspbaimage=dspba_prim.jpg  text=disp('min');  style=Optimised  visibilities=8+2^17  functionExpr=min  advOptions=[]  version=20121130
  MinMax1 : DSPBAPrim/MinMax  primtype=minmaxfunc  nInputs=2  nOutputs=1  omode=Specify via dialog  otype=constOTypeIn  scale=constScaleIn  rndmethod=Unbiased  factor=1  satmethod=Symmetric  shift_vec=[0 1 2 -1]  value=0  inPortNames=[' '; ' ';]  outPortNames=[' ']  dspbaimage=dspba_prim.jpg  text=disp('min');  style=Optimised  visibilities=8+2^17  functionExpr=max  advOptions=[]  version=20121130
  Sub : DSPBAPrim/Sub  primtype=sub  nInputs=2  nOutputs=1  omode=Inherit via internal rule  otype=sfix(16)  scale=2^-15  rndmethod=Unbiased  factor=1  satmethod=Symmetric  shift_vec=[0 1 2 -1]  value=0  inPortNames=['+'; '-';]  outPortNames=[' ']  dspbaimage=dspba_prim.jpg  text=fprintf('-');  style=Optimised  visibilities=8  floatRounding=correct  advOptions=[]  version=20130115
  const1 : DSPBAPrim/Const  primtype=const  nInputs=0  nOutputs=1  omode=Specify via dialog  otype=constOTypeIn  scale=constScaleIn  rndmethod=Unbiased  factor=1  satmethod=Symmetric  shift_vec=[0 1 2 -1]  value=0  inPortNames=['+'; '+';]  outPortNames=[' ']  dspbaimage=dspba_prim.jpg  text=fprintf('%s', num2str(value));  style=Optimised  visibilities=8 + 1024  floatPrecision=float32_m23  version=20120820
  Out1 : Outport
  wires:
  MinMax/1 -> MinMax1/1
  MinMax1/1 -> Out1/1
  Sub/1 -> MinMax1/2
  In1/1 -> MinMax/2
  const1/1 -> Sub/1
  limit/1 -> Sub/2, MinMax/1

== system foc_blocks/FL_fixp16/Fixed Saturate2 ==
  In1 : Inport
  limit : Inport  Port=2
  MinMax : DSPBAPrim/MinMax  primtype=minmaxfunc  nInputs=2  nOutputs=1  omode=Specify via dialog  otype=constOTypeIn  scale=constScaleIn  rndmethod=Unbiased  factor=1  satmethod=Symmetric  shift_vec=[0 1 2 -1]  value=0  inPortNames=[' '; ' ';]  outPortNames=[' ']  dspbaimage=dspba_prim.jpg  text=disp('min');  style=Optimised  visibilities=8+2^17  functionExpr=min  advOptions=[]  version=20121130
  MinMax1 : DSPBAPrim/MinMax  primtype=minmaxfunc  nInputs=2  nOutputs=1  omode=Specify via dialog  otype=constOTypeIn  scale=constScaleIn  rndmethod=Unbiased  factor=1  satmethod=Symmetric  shift_vec=[0 1 2 -1]  value=0  inPortNames=[' '; ' ';]  outPortNames=[' ']  dspbaimage=dspba_prim.jpg  text=disp('min');  style=Optimised  visibilities=8+2^17  functionExpr=max  advOptions=[]  version=20121130
  Sub : DSPBAPrim/Sub  primtype=sub  nInputs=2  nOutputs=1  omode=Inherit via internal rule  otype=sfix(16)  scale=2^-15  rndmethod=Unbiased  factor=1  satmethod=Symmetric  shift_vec=[0 1 2 -1]  value=0  inPortNames=['+'; '-';]  outPortNames=[' ']  dspbaimage=dspba_prim.jpg  text=fprintf('-');  style=Optimised  visibilities=8  floatRounding=correct  advOptions=[]  version=20130115
  const1 : DSPBAPrim/Const  primtype=const  nInputs=0  nOutputs=1  omode=Specify via dialog  otype=constOTypeIn  scale=constScaleIn  rndmethod=Unbiased  factor=1  satmethod=Symmetric  shift_vec=[0 1 2 -1]  value=0  inPortNames=['+'; '+';]  outPortNames=[' ']  dspbaimage=dspba_prim.jpg  text=fprintf('%s', num2str(value));  style=Optimised  visibilities=8 + 1024  floatPrecision=float32_m23  version=20120820
  Out1 : Outport
  wires:
  limit/1 -> MinMax/1, Sub/2
  const1/1 -> Sub/1
  In1/1 -> MinMax/2
  Sub/1 -> MinMax1/2
  MinMax1/1 -> Out1/1
  MinMax/1 -> MinMax1/1

== system foc_blocks/FL_fixp16/PI_Ctrl_D_DSPBA ==
  note: Ki
  note: Kp
  note: Saturate Limit
  note: Integral Output
  note: Integral Input
  note: Correction Output
  note: Saturate
  note: Saturate
  note: Integral Gain
  note: Proportional Gain
  note: Error Input
  note: Simple Proportional + Integral (PI) Controller
  PI_in : Inport
  Integral_in : Inport  Port=2
  Kp_in : Inport  Port=3
  Ki_in : Inport  Port=4
  Add1 : DSPBAPrim/Add  primtype=add  nInputs=evalAionMaskParam(gcb,'value',1)  nOutputs=1  omode=Inherit via internal rule with word growth  otype=sfix(16)  scale=2^-15  rndmethod=Unbiased  factor=1  satmethod=Symmetric  shift_vec=[0 1 2 -1]  value=2  inPortNames=[' '; ' ';]  outPortNames=[' ']  dspbaimage=dspba_prim.jpg  text=fprintf('+');  style=Optimised  visibilities=1032  genFPC=off  floatRounding=correct  advOptions=[]  version=20130821
  Add4 : DSPBAPrim/Add  primtype=add  nInputs=evalAionMaskParam(gcb,'value',1)  nOutputs=1  omode=Inherit via internal rule with word growth  otype=sfix(16)  scale=2^-15  rndmethod=Unbiased  factor=1  satmethod=Symmetric  shift_vec=[0 1 2 -1]  value=2  inPortNames=[' '; ' ';]  outPortNames=[' ']  dspbaimage=dspba_prim.jpg  text=fprintf('+');  style=Optimised  visibilities=1032  genFPC=off  floatRounding=correct  advOptions=[]  version=20130821
  Altera DSP Builder Advanced : AlteraGenericMotorLibrary/FP_Cur_Ctrl_DSPBA/Altera DSP Builder Advanced  SystemSampleTime=-1  VariantActivationTime=update diagram  Latency=0  AutoFrameSizeCalculation=off
  Fixed Saturate1 : Subsystem
  Fixed Saturate2 : Subsystem
  Mult : DSPBAPrim/Mult  primtype=mult  nInputs=2  nOutputs=1  omode=Specify via dialog  otype=constOTypeMult  scale=constScaleIn  rndmethod=Unbiased  factor=1  satmethod=Symmetric  shift_vec=[0 1 2 -1]  value=0  inPortNames=[' '; ' ';]  outPortNames=[' ']  dspbaimage=dspba_prim.jpg  text=fprintf('X');  style=Optimised  visibilities=8  floatPrecision=float32_m23  floatRounding=correct  advOptions=[]  version=20130115
  Mult1 : DSPBAPrim/Mult  primtype=mult  nInputs=2  nOutputs=1  omode=Specify via dialog  otype=constOTypeMult  scale=constScaleIn  rndmethod=Unbiased  factor=1  satmethod=Symmetric  shift_vec=[0 1 2 -1]  value=0  inPortNames=[' '; ' ';]  outPortNames=[' ']  dspbaimage=dspba_prim.jpg  text=fprintf('X');  style=Optimised  visibilities=8  floatPrecision=float32_m23  floatRounding=correct  advOptions=[]  version=20130115
  const1 : DSPBAPrim/Const  primtype=const  nInputs=0  nOutputs=1  omode=Specify via dialog  otype=constOTypeIn  scale=constScaleIn  rndmethod=Unbiased  factor=1  satmethod=Symmetric  shift_vec=[0 1 2 -1]  value=0.95*2^(constwordlengthIn-constfractionlengthIn-1)  inPortNames=['+'; '+';]  outPortNames=[' ']  dspbaimage=dspba_prim.jpg  text=fprintf('%s', num2str(value));  style=Optimised  visibilities=8 + 1024  floatPrecision=float32_m23  version=20120820
  PI_out : Outport
  I_out : Outport  Port=2
  wires:
  Ki_in/1 -> Mult1/2
  Kp_in/1 -> Mult/2
  Integral_in/1 -> Add4/2
  Add4/1 -> Fixed Saturate2/1(In1)
  Mult1/1 -> Add4/1
  Fixed Saturate2/1(Out1) -> I_out/1, Add1/2
  Mult/1 -> Add1/1
  PI_in/1 -> Mult/1, Mult1/1
  Add1/1 -> Fixed Saturate1/1(In1)
  Fixed Saturate1/1(Out1) -> PI_out/1
  const1/1 -> Fixed Saturate1/2(limit), Fixed Saturate2/2(limit)

== system foc_blocks/FL_fixp16/PI_Ctrl_D_DSPBA1 ==
  note: Simple Proportional + Integral (PI) Controller
  note: Error Input
  note: Proportional Gain
  note: Integral Gain
  note: Saturate
  note: Saturate
  note: Correction Output
  note: Integral Input
  note: Integral Output
  note: Saturate Limt
  note: Kp
  note: Ki
  PI_in : Inport
  Integral_in : Inport  Port=2
  Kp_in : Inport  Port=3
  Ki_in : Inport  Port=4
  Add1 : DSPBAPrim/Add  primtype=add  nInputs=evalAionMaskParam(gcb,'value',1)  nOutputs=1  omode=Inherit via internal rule with word growth  otype=sfix(16)  scale=2^-15  rndmethod=Unbiased  factor=1  satmethod=Symmetric  shift_vec=[0 1 2 -1]  value=2  inPortNames=[' '; ' ';]  outPortNames=[' ']  dspbaimage=dspba_prim.jpg  text=fprintf('+');  style=Optimised  visibilities=1032  genFPC=off  floatRounding=correct  advOptions=[]  version=20130821
  Add4 : DSPBAPrim/Add  primtype=add  nInputs=evalAionMaskParam(gcb,'value',1)  nOutputs=1  omode=Inherit via internal rule with word growth  otype=sfix(16)  scale=2^-15  rndmethod=Unbiased  factor=1  satmethod=Symmetric  shift_vec=[0 1 2 -1]  value=2  inPortNames=[' '; ' ';]  outPortNames=[' ']  dspbaimage=dspba_prim.jpg  text=fprintf('+');  style=Optimised  visibilities=1032  genFPC=off  floatRounding=correct  advOptions=[]  version=20130821
  Altera DSP Builder Advanced : AlteraGenericMotorLibrary/FP_Cur_Ctrl_DSPBA/Altera DSP Builder Advanced  SystemSampleTime=-1  VariantActivationTime=update diagram  Latency=0  AutoFrameSizeCalculation=off
  Fixed Saturate1 : Subsystem
  Fixed Saturate2 : Subsystem
  Mult : DSPBAPrim/Mult  primtype=mult  nInputs=2  nOutputs=1  omode=Specify via dialog  otype=constOTypeMult  scale=constScaleIn  rndmethod=Unbiased  factor=1  satmethod=Symmetric  shift_vec=[0 1 2 -1]  value=0  inPortNames=[' '; ' ';]  outPortNames=[' ']  dspbaimage=dspba_prim.jpg  text=fprintf('X');  style=Optimised  visibilities=8  floatPrecision=float32_m23  floatRounding=correct  advOptions=[]  version=20130115
  Mult1 : DSPBAPrim/Mult  primtype=mult  nInputs=2  nOutputs=1  omode=Specify via dialog  otype=constOTypeMult  scale=constScaleIn  rndmethod=Unbiased  factor=1  satmethod=Symmetric  shift_vec=[0 1 2 -1]  value=0  inPortNames=[' '; ' ';]  outPortNames=[' ']  dspbaimage=dspba_prim.jpg  text=fprintf('X');  style=Optimised  visibilities=8  floatPrecision=float32_m23  floatRounding=correct  advOptions=[]  version=20130115
  const1 : DSPBAPrim/Const  primtype=const  nInputs=0  nOutputs=1  omode=Specify via dialog  otype=constOTypeIn  scale=constScaleIn  rndmethod=Unbiased  factor=1  satmethod=Symmetric  shift_vec=[0 1 2 -1]  value=0.95*2^(constwordlengthIn-constfractionlengthIn-1)  inPortNames=['+'; '+';]  outPortNames=[' ']  dspbaimage=dspba_prim.jpg  text=fprintf('%s', num2str(value));  style=Optimised  visibilities=8 + 1024  floatPrecision=float32_m23  version=20120820
  PI_out : Outport
  I_out : Outport  Port=2
  wires:
  Fixed Saturate1/1(Out1) -> PI_out/1
  Add1/1 -> Fixed Saturate1/1(In1)
  PI_in/1 -> Mult1/1, Mult/1
  Mult/1 -> Add1/1
  Fixed Saturate2/1(Out1) -> Add1/2, I_out/1
  Mult1/1 -> Add4/1
  Add4/1 -> Fixed Saturate2/1(In1)
  Integral_in/1 -> Add4/2
  Kp_in/1 -> Mult/2
  Ki_in/1 -> Mult1/2
  const1/1 -> Fixed Saturate2/2(limit), Fixed Saturate1/2(limit)
